simulink model "LED_Switch_Model"  (R2025a)
settings: Solver=FixedStepDiscrete  StartTime=0.0  StopTime=20  FixedStep=1  RelTol=1e-3
libraries: simulink x3
settings Model: Creator=mahij  LastModifiedBy=mahij

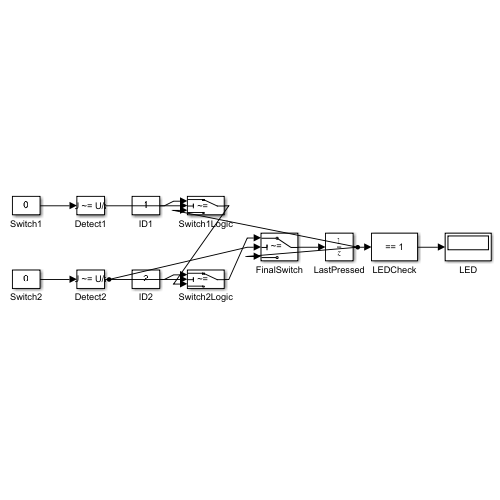
[thumbnail: Simulink's stored preview of the top-level diagram]
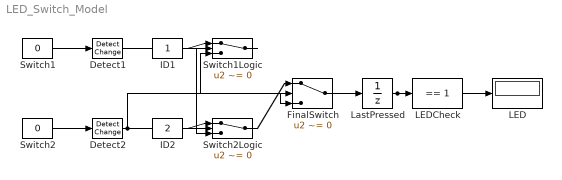
== system LED_Switch_Model ==
  Detect1 : simulink/Logic and Bit Operations/Detect Change  vinit=0  OutDataTypeStr=boolean
  Detect2 : simulink/Logic and Bit Operations/Detect Change  vinit=0  OutDataTypeStr=boolean
  FinalSwitch : Switch  Criteria=u2 ~= 0  Threshold=0.5  SaturateOnIntegerOverflow=off  InputSameDT=off
  ID1 : Constant
  ID2 : Constant  Value=2
  LED : Display
  LEDCheck : simulink/Logic and Bit Operations/Compare To Constant  relop===  const=1  OutDataTypeStr=boolean
  LastPressed : UnitDelay  HasFrameUpgradeWarning=on
  Switch1 : Constant  Value=0
  Switch1Logic : Switch  Criteria=u2 ~= 0  Threshold=0.5  SaturateOnIntegerOverflow=off  InputSameDT=off
  Switch2 : Constant  Value=0
  Switch2Logic : Switch  Criteria=u2 ~= 0  Threshold=0.5  SaturateOnIntegerOverflow=off  InputSameDT=off
  wires:
  Switch1/1 -> Detect1/1
  Switch2/1 -> Detect2/1
  ID1/1 -> Switch1Logic/1
  Detect1/1 -> Switch1Logic/2
  LastPressed/1 -> Switch1Logic/3, FinalSwitch/3, LEDCheck/1
  ID2/1 -> Switch2Logic/1
  Detect2/1 -> Switch2Logic/2, FinalSwitch/2
  Switch1Logic/1 -> Switch2Logic/3
  Switch2Logic/1 -> FinalSwitch/1
  FinalSwitch/1 -> LastPressed/1
  LEDCheck/1 -> LED/1
